simulink model "R_Mode_v1"  (R2020a)
settings: Solver=FixedStepAuto  StartTime=0.0  StopTime=10.0  FixedStep=1e-3  RelTol=1e-3  EnableMultiTasking=on
undefined symbols (not defined in the file): D0, D1, D10, D11, D12, D13, D2, D3, D4, D5, D6, D7, D8, D9, PTA0, PTA1, PTA2, PTB23, PTB9, PTC16, PTC17, PTC2, PTC3, PTC4, PTD0, PTD1, PTD2, PTD3
libraries: frdmk64flib x23
settings Model: ExtModeTrigDuration=5  Creator=forre  LastModifiedBy=forre
settings OptimizationCC: EnhancedBackFolding=on  PassReuseOutputArgsAs=Individual arguments  ZeroExternalMemoryAtStartup=off  ZeroInternalMemoryAtStartup=off  MaxStackSize=64  OptimizeBlockOrder=speed  DifferentSizesBufferReuse=on  OptimizationCustomize=off  EfficientTunableParamExpr=on
settings DebuggingCC: ParameterTunabilityLossMsg=error
settings HardwareCC: ProdBitPerPointer=32  ProdBitPerSizeT=32  ProdBitPerPtrDiffT=32  ProdLargestAtomicInteger=Long  ProdLargestAtomicFloat=Double  ProdWordSize=32  ProdHWDeviceType=ARM Compatible->ARM Cortex
settings SFSimCC: MATLABDynamicMemAlloc=off
settings RTWCC: SystemTargetFile=ert.tlc  HardwareBoard=NXP FRDM-K64F  TemplateMakefile=ert_default_tmf  Toolchain=GNU Tools for ARM Embedded Processors
settings CodeAppCC: ForceParamTrailComments=on  IgnoreCustomStorageClasses=off  OperatorAnnotations=on  SimulinkDataObjDesc=on  SFDataObjDesc=on  InsertBlockDesc=on

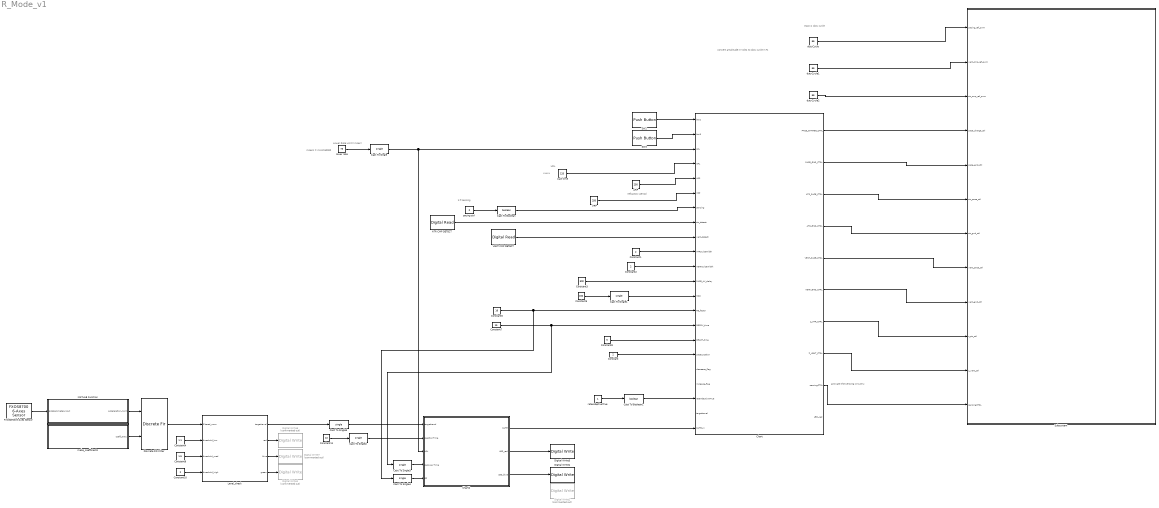
== system R_Mode_v1 ==
  note: convert amplitude in Volts to duty cycle in %
  note: *****
  note: msecs = mins*60000
  note: URL
  note: refractory period
  note: Lower Rate Limit (msec)
  note: activate the sensing circuitry.
  note: input = duty cycle
  note: 1 if sensing
  ARP : Constant  Value=250
  ATR CMP DETECT : frdmk64flib/Digital Read  Whichpin=PTC16 (D0)  SampleTime=-1
  Cast To Boolean : DataTypeConversion  OutDataTypeStr=boolean
  Cast To Boolean1 : DataTypeConversion  OutDataTypeStr=boolean
  Cast To Single{,1..5} (6 alike) : DataTypeConversion  OutDataTypeStr=single
  Chart : Stateflow chart  TreatAsAtomicUnit=on
  Chart2 : Stateflow chart  TreatAsAtomicUnit=on
  Constant : Constant  Value=2  OutDataTypeStr=double
  Constant1 : Constant  Value=2
  Constant10 : Constant  Value=2  OutDataTypeStr=double
  Constant11 : Constant  Value=10  OutDataTypeStr=double
  Constant2 : Constant  Value=2
  Constant3 : Constant  Value=500
  Constant4 : Constant  Value=1.1  OutDataTypeStr=double
  Constant5 : Constant  Value=150  OutDataTypeStr=double
  Constant6 : Constant  Value=16  OutDataTypeStr=double
  Constant7 : Constant  Value=15  OutDataTypeStr=double
  Constant8 : Constant  Value=5  OutDataTypeStr=double
  Constant9 : Constant  Value=1.5  OutDataTypeStr=double
  Digital Write1 : frdmk64flib/Digital Write  Commented=on  Whichpin=GREEN_LED
  Digital Write2 : frdmk64flib/Digital Write  Commented=on  Whichpin=GREEN_LED
  Digital Write3 : frdmk64flib/Digital Write  Whichpin=RED_LED
  Digital Write4 : frdmk64flib/Digital Write  Whichpin=BLUE_LED
  Digital Write6 : frdmk64flib/Digital Write  Commented=on  Whichpin=RED_LED
  Digital Write7 : frdmk64flib/Digital Write  Commented=on  Whichpin=BLUE_LED
  Discrete FIR Filter : DiscreteFir  CoefSource=Input port  Coefficients=[0.05, 0.05, 0.05,0.05, 0.05, 0.05, 0.05, 0.05,0.05, 0.05,0.05, 0.05, 0.05,0.05, 0.05, 0.05, 0.05, 0.05,0.05, 0.05]
      settings: InputPortMap=u0,u1
  FXOS8700 6-Axes Sensor : frdmk64flib/FXOS8700 6-Axes Sensor  Activesensor=Accelerometer only  ODR=800Hz  HybridODR=400Hz  Accelfullrange=-2g to +2g  SampleTime=-1
  Level_check : MATLAB Function  TreatAsAtomicUnit=on
  MATLAB Function : MATLAB Function  TreatAsAtomicUnit=on
  SW2 : frdmk64flib/Push Button  Whichswitch=SW2  SampleTime1=-1
  SW3 : frdmk64flib/Push Button  Whichswitch=SW3  SampleTime1=-1
  Subsystem : Subsystem
  VENT CMP DETECT : frdmk64flib/Digital Read  Whichpin=PTC17 (D1)  SampleTime=-1
  VRP : Constant  Value=250
  dutyCycle : Constant  Value=66
  dutyCycle1 : Constant  Value=66
  dutyCycle2 : Constant  Value=66
  lower rate : Constant  Value=75
  make_coefficients : MATLAB Function  TreatAsAtomicUnit=on
  pacing ctrl : Constant  Value=0
  rateAdaptiveTrue : Constant
  wait time : Constant  Value=120
  wires:
  dutyCycle/1 -> Subsystem/1(pacing_ref_pwm)
  SW2/1 -> Chart/1(btn2)
  Chart/4(ATR_GND_CTRL) -> Subsystem/7(atr_gnd_ctrl)
  Constant1/1 -> Chart/10(ATRpulseWidth)
  Chart/3(ATR_PACE_CTRL) -> Subsystem/6(atr_pace_ctrl)
  Chart/1(PACE_CHARGE_CTRL) -> Subsystem/4(pace_charge_ctrl)
  Chart/2(PACE_GND_CTRL) -> Subsystem/5(pace_gnd_ctrl)
  lower rate/1 -> Cast To Single/1
  Chart/5(VENT_PACE_CTRL) -> Subsystem/8(vent_pace_ctrl)
  Chart/6(VENT_GND_CTRL) -> Subsystem/9(vent_gnd_ctrl)
  Chart/7(Z_ATR_CTRL) -> Subsystem/10(z_atr_ctrl)
  Chart/8(Z_VENT_CTRL) -> Subsystem/11(" z_vent_ctrl")
  pacing ctrl/1 -> Cast To Boolean/1
  ATR CMP DETECT/1 -> Chart/8(atr_detect)
  VENT CMP DETECT/1 -> Chart/9(vent_detect)
  dutyCycle1/1 -> Subsystem/2(vent_cmp_ref_pwm)
  dutyCycle2/1 -> Subsystem/3(atr_cmp_ref_pwm)
  Chart/9(sensingCTRL) -> Subsystem/12(sensingCTRL)
  Cast To Boolean/1 -> Chart/7(sensing)
  Chart2/3(LED_blue) -> Digital Write4/1
  SW3/1 -> Chart/2(btn3)
  wait time/1 -> Chart/4(URL)
  ARP/1 -> Chart/5(ARP)
  VRP/1 -> Chart/6(VRP)
  Constant2/1 -> Chart/11(VENTpulseWidth)
  Constant/1 -> Chart/17(paceLocation)
  Constant3/1 -> Chart/12(PACE_AV_delay)
  Constant5/1 -> Cast To Single1/1
  Constant6/1 -> Chart/14(RE_factor), Cast To Single4/1
  Constant7/1 -> Chart/15(RECOV_time), Cast To Single3/1
  Constant8/1 -> Chart/16(REACT_time)
  Cast To Boolean1/1 -> Chart/20(rateAdaptiveTrue)
  rateAdaptiveTrue/1 -> Cast To Boolean1/1
  Chart2/1(RATE) -> Chart/22(RATE_in)
  Cast To Single/1 -> Chart/3(LRL), Chart2/3(LRL)
  Constant11/1 -> Cast To Single2/1
  Cast To Single1/1 -> Chart/13(MSR)
  Cast To Single2/1 -> Chart2/2(reactionTime)
  Cast To Single3/1 -> Chart2/4(recoveryTime)
  Cast To Single4/1 -> Chart2/5(RF)
  Chart2/2(LED_red) -> Digital Write3/1
  FXOS8700 6-Axes Sensor/1 -> MATLAB Function/1(accelerometer_input)
  Constant4/1 -> Level_check/2(threshold_low)
  Constant10/1 -> Level_check/4(threshold_high)
  Constant9/1 -> Level_check/3(threshold_med)
  Level_check/1(targetLevel) -> Cast To Single5/1
  MATLAB Function/1(acceleration_norm) -> Discrete FIR Filter/1
  Discrete FIR Filter/1 -> Level_check/1(filtered_norm)
  Level_check/2(red) -> Digital Write6/1
  Level_check/3(blue) -> Digital Write7/1
  Level_check/4(green) -> Digital Write1/1
  Cast To Single5/1 -> Chart2/1(targetLevel)
  make_coefficients/1(coeff_array) -> Discrete FIR Filter/2

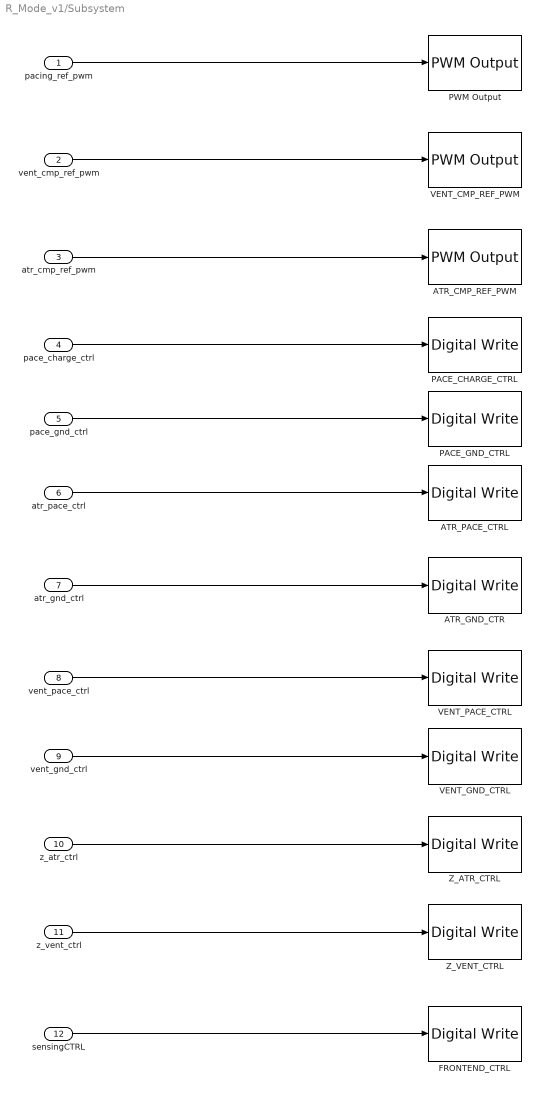
== system R_Mode_v1/Subsystem ==
  pacing_ref_pwm : Inport
  vent_cmp_ref_pwm : Inport  Port=2
  atr_cmp_ref_pwm : Inport  Port=3
  pace_charge_ctrl : Inport  Port=4
  pace_gnd_ctrl : Inport  Port=5
  atr_pace_ctrl : Inport  Port=6
  atr_gnd_ctrl : Inport  Port=7
  vent_pace_ctrl : Inport  Port=8
  vent_gnd_ctrl : Inport  Port=9
  z_atr_ctrl : Inport  Port=10
  " z_vent_ctrl" : Inport  Port=11
  sensingCTRL : Inport  Port=12
  ATR_CMP_REF_PWM : frdmk64flib/PWM Output  Whichpin=PTC2 (D6)  InitialFrequency=2000  InitialDutyCycle=50
  ATR_GND_CTR : frdmk64flib/Digital Write  Whichpin=PTD2 (D11)
  ATR_PACE_CTRL : frdmk64flib/Digital Write  Whichpin=PTA0 (D8)
  FRONTEND_CTRL : frdmk64flib/Digital Write  Whichpin=PTD1 (D13)
  PACE_CHARGE_CTRL : frdmk64flib/Digital Write  Whichpin=PTB9 (D2)
  PACE_GND_CTRL : frdmk64flib/Digital Write  Whichpin=PTD0 (D10)
  PWM Output : frdmk64flib/PWM Output  Whichpin=PTA2 (D5)  InitialFrequency=2000  InitialDutyCycle=50
  VENT_CMP_REF_PWM : frdmk64flib/PWM Output  Whichpin=PTA1 (D3)  InitialFrequency=2000  InitialDutyCycle=50
  VENT_GND_CTRL : frdmk64flib/Digital Write  Whichpin=PTD3 (D12)
  VENT_PACE_CTRL : frdmk64flib/Digital Write  Whichpin=PTC4 (D9)
  Z_ATR_CTRL : frdmk64flib/Digital Write  Whichpin=PTB23 (D4)
  Z_VENT_CTRL : frdmk64flib/Digital Write  Whichpin=PTC3 (D7)
  wires:
  pace_gnd_ctrl/1 -> PACE_GND_CTRL/1
  atr_pace_ctrl/1 -> ATR_PACE_CTRL/1
  pace_charge_ctrl/1 -> PACE_CHARGE_CTRL/1
  atr_gnd_ctrl/1 -> ATR_GND_CTR/1
  vent_pace_ctrl/1 -> VENT_PACE_CTRL/1
  vent_gnd_ctrl/1 -> VENT_GND_CTRL/1
  z_atr_ctrl/1 -> Z_ATR_CTRL/1
  " z_vent_ctrl"/1 -> Z_VENT_CTRL/1
  sensingCTRL/1 -> FRONTEND_CTRL/1
  pacing_ref_pwm/1 -> PWM Output/1
  vent_cmp_ref_pwm/1 -> VENT_CMP_REF_PWM/1
  atr_cmp_ref_pwm/1 -> ATR_CMP_REF_PWM/1

== stateflow chart R_Mode_v1/Chart ==
  note: IF target level > previous level
  note: target Level = LEVEL
  note: if level = 0
      | RATE = LRL
      |
      | if level = 1
      | RATE = LRL + ResponseFactor
      |
      | if level = 2
      | RATE = LRL + 2*ResponseFactor
      |
      | if level = 3
      | RATE = LRL + 3*ResponseFactor
  state INCREMENT_VENT [commented out]
    entry:
    incrementTime=reactionTime/((TargetLevel - PreviousLevel)*RF);
    % time/BPM increase
  note: incrementTime=reactionTime/((TargetLevel - PreviousLevel)*RF)
  state SENSING_VENT_TRUE
    entry:
    sensingCTRL = true;
  note: for VOO,VVI, so it don't go to REACTION_V and RECOVERY_V
  note: ventPflag = true
  state adaptRATE_vent
    % RE factor need to time a rate (unit ppm)
    %it is depend on LRL and MSR values
    %RATE_out = RATE
    RATE = RATE_in;
  note: new Idea!
      |
      | secPerPace = msecPerPace/1000
      |
      | reactionTime/secPerPace = %of increase per cycle
  note: no more change in RATE needed
  note: eg if reactionTIme = 10 and RATE = 60 BPM
      | 10/1 =10
      | incrementAmount = (targetLevel-previousLevel)*RF/10
      |
      | so each cycle RATE = RATE + incrementAmount
  state VENT_CHARGING_AND_DISCHARGE
    entry:
    % for this state paceLocation = 1
    %begin charge and discharge cycle for ventricle
    msecPerPace = 60000.0/RATE/2; %new value in msec
    sensingCTRL = sensing; %enables the sensing circuitry if sensing = 1. Controled by input "sensing"
    ATR_PACE_CTRL = false;
    VENT_PACE_CTRL = false;
    PACE_CHARGE_CTRL = true;
    PACE_GND_CTRL = true;
    Z_VENT_CTRL = false;
    Z_ATR_CTRL = false
    VENT_GND_CTRL = true;
    ATR_GND_CTRL = false;
  state VENT_PACING
    entry:
    % pace ventricle
    PACE_CHARGE_CTRL = false;
    PACE_GND_CTRL = true;
    VENT_PACE_CTRL = true;
    VENT_GND_CTRL = false;
    Z_VENT_CTRL = false;
    Z_ATR_CTRL = false;
    ATR_GND_CTRL = false;
    ATR_PACE_CTRL = false;
    sensingCTRL = sensing; %enables the sensing circuitry if sensing = 1. Controled by input "sensing"
    %VENT_P_flag = true; %pacing flag for V modes
    %recovery
    %recoveryTime_remaining = recoveryTime_remaining - (msecPerPace-VENTpulseWidth)
    LED_red=false;
  note: reactionTime_remaining
  note: recoveryTime_remaining
  note: beat sensed
  note: R_MODE
  note: VENT PACING
  note: SWITCH TO VOO,VVI,VOOR,VVIR
  state RECOVERY_V [commented out]
    RATE = RATE - LEVEL*RE_factor
    % RE factor need to time a rate (unit ppm)
    %it is depend on LRL and MSR values
  state REACTION_V [commented out]
    RATE = RATE + LEVEL*RE_factor;
    % RE factor need to time a rate (unit ppm)
    %it is depend on LRL and MSR values
  note: SWITCH TO AOO, AAI,AOOR,AAIR
  state ATR_PACING [commented out]
    entry:
    % pace atrium
    PACE_GND_CTRL = true;
    VENT_PACE_CTRL = false;
    VENT_GND_CTRL = false;
    Z_VENT_CTRL = false;
    Z_ATR_CTRL = false;
    ATR_GND_CTRL = false;
    ATR_PACE_CTRL = true;
    sensingCTRL = sensing; %enables the sensing circuitry if sensing = 1. Controled by input "sensing"
    ATR_P_flag = true; %pacing flag for V modes
  note: SWITCH TO DOO,DOOR
  state ATR_CHARGING_AND_DISCHARGE [commented out]
    entry:
    % for this state paceLocation = 0
    %begin charge and discharge cycle for atrium
    msecPerPace = 60000/RATE; %new value for pace timing with msec units
    sensingCTRL = sensing; %enables the sensing circuitry if sensing = 1. Controled by input "sensing"
    ATR_PACE_CTRL = false;
    VENT_PACE_CTRL = false;
    PACE_CHARGE_CTRL = true;
    PACE_GND_CTRL = true;
    Z_VENT_CTRL = false;
    Z_ATR_CTRL = false;
    VENT_GND_CTRL = false;
    ATR_GND_CTRL = true;
  note: R_MODE
  note: ATR PACING
  note: SWITCH TO VOO,VVI,VOOR,VVIR
  state SENSING_ATR_TRUE [commented out]
    entry:
    sensingCTRL = true;
  note: beat sensed
  note: SWITCH TO DOO,DOOR
  state RECOVERY_V1 [commented out]
    RATE = RATE - LEVEL*RE_factor
    % RE factor need to time a rate (unit ppm)
    %it is depend on LRL and MSR values
  note: SWITCH TO AOO, AAI,AOOR,AAIR
  state REACTION_V1 [commented out]
    RATE = RATE + LEVEL*RE_factor;
    % RE factor need to time a rate (unit ppm)
    %it is depend on LRL and MSR values
  state DUAL_ATR_CHARGING_AND_DISCHARGE [commented out]
    entry:
    msecPerPace = 60000/RATE;
    % for this state paceLocation = 3
    %begin charge and discharge cycle for atrium
    ATR_PACE_CTRL = false;
    VENT_PACE_CTRL = false;
    PACE_CHARGE_CTRL = true;
    PACE_GND_CTRL = true;
    Z_VENT_CTRL = false;
    Z_ATR_CTRL = false;
    VENT_GND_CTRL = false;
    ATR_GND_CTRL = true;
  state DUAL_ATR_PACING [commented out]
    entry:
    % pace atrium
    PACE_GND_CTRL = true;
    VENT_PACE_CTRL = false;
    VENT_GND_CTRL = false;
    Z_VENT_CTRL = false;
    Z_ATR_CTRL = false;
    ATR_GND_CTRL = false;
    ATR_PACE_CTRL = true;
    AP_flag = true; % rise to true when Atrium have a pace
  note: DOO,DOOR
  state DUAL_VENT_PACING [commented out]
    entry:
    % pace ventricle
    PACE_GND_CTRL = true;
    VENT_PACE_CTRL = true;
    VENT_GND_CTRL = false;
    Z_VENT_CTRL = false;
    Z_ATR_CTRL = false;
    ATR_GND_CTRL = false;
    ATR_PACE_CTRL = false;
    sensingCTRL = sensing; %enables the sensing circuitry if sensing = 1. Controled by input "sensing"
    AP_flag = false;
  state DUAL_VENT_CHARGING_AND_DISCHARGE [commented out]
    entry:
    %begin charge and discharge cycle for ventricle
    msecPerPace = 60000/RATE; %new value in msec
    sensingCTRL = sensing; %enables the sensing circuitry if sensing = 1. Controled by input "sensing"
    ATR_PACE_CTRL = false;
    VENT_PACE_CTRL = false;
    PACE_CHARGE_CTRL = true;
    PACE_GND_CTRL = true;
    Z_VENT_CTRL = false;
    Z_ATR_CTRL = false
    VENT_GND_CTRL = true;
    ATR_GND_CTRL = false;
  INCREMENT_VENT -> INCREMENT_VENT [commented out] : after(incrementTime)[reactionTime_remaining>0]{RATE=RATE+1;reactionTime_remaining-incrementTime;}
  (junction 296) -> VENT_CHARGING_AND_DISCHARGE [order 1] : [rateAdaptiveTrue == false]{RATE=LRL}
  VENT_CHARGING_AND_DISCHARGE -> SENSING_VENT_TRUE [order 2] : after((VRP-VENTpulseWidth),msec)[sensing && (vent_detect || btn3)]
  SENSING_VENT_TRUE -> VENT_CHARGING_AND_DISCHARGE : after(VENTpulseWidth, msec)
  INCREMENT_VENT -> INCREMENT_VENT [commented out] : [reactionTime_remaining <= 0]{previousLevel = LEVEL}
  VENT_PACING -> (junction 296) : after(VENTpulseWidth, msec)
  (junction 296) -> adaptRATE_vent [order 2] : [rateAdaptiveTrue == true]
  adaptRATE_vent -> (junction 386) [commented out] : [(decrease_flag == false && increase_flag == false)]
  adaptRATE_vent -> adaptRATE_vent [commented out] : [increase_flag == true && (RATE < MSR)]{RATE = RATE_in;LED_red=true;}
  (junction 386) -> VENT_CHARGING_AND_DISCHARGE [order 1] : [RATE< LRL]{RATE = LRL}
  adaptRATE_vent -> (junction 386)
  (junction 386) -> VENT_CHARGING_AND_DISCHARGE [order 2] : [RATE>MSR]{RATE=MSR}
  (junction 386) -> VENT_CHARGING_AND_DISCHARGE [order 3]
  (default) -> VENT_CHARGING_AND_DISCHARGE : {RATE=LRL;LED_red=false;previousLevel = 0;}
  adaptRATE_vent -> adaptRATE_vent [commented out] : [decrease_flag == true && (RATE > LRL)]{RATE = RATE_in}
  VENT_CHARGING_AND_DISCHARGE -> DUAL_ATR_CHARGING_AND_DISCHARGE [commented out] : [(paceLocation == 3) || (paceLocation == 6)]{RATE=LRL}
  (junction 290) -> VENT_CHARGING_AND_DISCHARGE [commented out]
  DUAL_ATR_CHARGING_AND_DISCHARGE -> (junction 290) [commented out] : [(paceLocation == 2) || (paceLocation == 4)]{RATE=LRL}
  ATR_CHARGING_AND_DISCHARGE -> (junction 290) [commented out] : [(paceLocation == 2) || (paceLocation == 4)]{RATE=LRL}
  VENT_CHARGING_AND_DISCHARGE -> VENT_PACING [order 1] : after((msecPerPace-VENTpulseWidth), msec)
  RECOVERY_V -> ? [commented out] : after(((RECOV_time/RE_factor)*60),sec){VENT_P_flag = false}
  VENT_CHARGING_AND_DISCHARGE -> (junction 361) [commented out] : [(paceLocation==4)&&(VENT_P_flag== true)]
  (junction 361) -> VENT_CHARGING_AND_DISCHARGE [commented out] : [increase_flag == false]{VENT_P_flag = false}
  (junction 322) -> VENT_CHARGING_AND_DISCHARGE [commented out] : [(RATE>=MSR)]{RATE=MSR,VENT_P_flag = false}
  REACTION_V -> VENT_CHARGING_AND_DISCHARGE [commented out] : after((REACT_time/RE_factor),sec){VENT_P_flag = false}
  VENT_CHARGING_AND_DISCHARGE -> ATR_CHARGING_AND_DISCHARGE [commented out] : [(paceLocation == 1)|| (paceLocation == 5)]{RATE=LRL,ATR_P_flag = false}
  (junction 366) -> ? [commented out] : [(RATE<=LRL)]{RATE = LRL,VENT_P_flag = false}
  (default) -> (junction 326) [commented out] : [(paceLocation==4)&&(VENT_P_flag== true)]
  (junction 326) -> ? [commented out] : [decrease_flag == false]{VENT_P_flag = false}
  (junction 361) -> (junction 322) [commented out] : [increase_flag == true]
  (junction 326) -> (junction 366) [commented out] : [decrease_flag == true]
  (junction 366) -> RECOVERY_V [commented out] : [(RATE>LRL)]
  (junction 322) -> REACTION_V [commented out] : [RATE<MSR]
  (junction 347) -> ATR_CHARGING_AND_DISCHARGE [commented out] : [paceLocation == 1]{ATR_P_flag = false}
  ATR_PACING -> (junction 347) [commented out] : after(ATRpulseWidth, msec)
  (junction 347) -> ATR_CHARGING_AND_DISCHARGE [commented out] : [paceLocation == 5]
  ATR_CHARGING_AND_DISCHARGE -> (junction 282) [commented out] : [(paceLocation == 3) || (paceLocation == 6)]{RATE=LRL}
  ATR_CHARGING_AND_DISCHARGE -> (junction 353) [commented out] : [ATR_P_flag == false]
  (junction 353) -> ATR_PACING [commented out] : after((msecPerPace-ATRpulseWidth), msec){PACE_CHARGE_CTRL = false;}
  RECOVERY_V1 -> ATR_CHARGING_AND_DISCHARGE [commented out] : after(((RECOV_time/RE_factor)*60),sec){ATR_P_flag = false}
  REACTION_V1 -> ATR_CHARGING_AND_DISCHARGE [commented out] : after((REACT_time/RE_factor),sec){ATR_P_flag = false}
  (junction 341) -> ATR_CHARGING_AND_DISCHARGE [commented out] : [RATE<=LRL]{RATE = LRL,ATR_P_flag = false}
  (junction 331) -> ATR_CHARGING_AND_DISCHARGE [commented out] : [LEVEL==0]{RATE = LRL,ATR_P_flag = false}
  ATR_CHARGING_AND_DISCHARGE -> (junction 341) [commented out] : [(paceLocation==5)&&(ATR_P_flag== true)]
  ATR_CHARGING_AND_DISCHARGE -> SENSING_ATR_TRUE [commented out] : after((ARP-ATRpulseWidth),msec)[sensing && (atr_detect || btn3)]
  SENSING_ATR_TRUE -> ATR_CHARGING_AND_DISCHARGE [commented out] : after(ATRpulseWidth, msec)
  DUAL_ATR_CHARGING_AND_DISCHARGE -> ATR_CHARGING_AND_DISCHARGE [commented out] : [(paceLocation == 1)|| (paceLocation == 5)]{RATE=LRL,ATR_P_flag == false}
  ATR_CHARGING_AND_DISCHARGE -> (junction 336) [commented out] : [(paceLocation==5)&&(ATR_P_flag== true)]
  (junction 336) -> ATR_CHARGING_AND_DISCHARGE [commented out] : [RATE>=MSR]{RATE=MSR,ATR_P_flag = false}
  (junction 341) -> RECOVERY_V1 [commented out] : [RATE>LRL]
  (junction 336) -> (junction 331) [commented out] : [RATE<MSR]
  (junction 331) -> REACTION_V1 [commented out] : [LEVEL>0]
  (junction 282) -> DUAL_ATR_CHARGING_AND_DISCHARGE [commented out] : {AP_flag == false}
  DUAL_ATR_CHARGING_AND_DISCHARGE -> DUAL_ATR_PACING [commented out] : [AP_flag == false]{PACE_CHARGE_CTRL = false;}
  DUAL_ATR_PACING -> DUAL_ATR_CHARGING_AND_DISCHARGE [commented out] : after( ATRpulseWidth, msec)
  DUAL_ATR_CHARGING_AND_DISCHARGE -> (junction 285) [commented out] : [AP_flag == true]
  (junction 285) -> DUAL_VENT_CHARGING_AND_DISCHARGE [commented out] : after(PACE_AV_delay-ATRpulseWidth,msec)
  (junction 288) -> DUAL_ATR_CHARGING_AND_DISCHARGE [commented out] : [AP_flag == false]
  DUAL_VENT_PACING -> DUAL_VENT_CHARGING_AND_DISCHARGE [commented out] : after((VENTpulseWidth), msec)
  DUAL_VENT_CHARGING_AND_DISCHARGE -> DUAL_VENT_PACING [commented out] : [AP_flag == true]{PACE_CHARGE_CTRL = false;}
  DUAL_VENT_CHARGING_AND_DISCHARGE -> (junction 288) [commented out] : after(msecPerPace-VENTpulseWidth-PACE_AV_delay,msec)
  data: PACE_CHARGE_CTRL output boolean; PACE_GND_CTRL output boolean; btn2 input boolean; btn3 input boolean; ATR_PACE_CTRL output boolean; ATR_GND_CTRL output boolean; LRL input single; URL input double; ARP input double; VRP input double; VENT_PACE_CTRL output boolean; VENT_GND_CTRL output boolean; Z_ATR_CTRL output boolean; Z_VENT_CTRL output boolean; sensing input boolean; atr_detect input boolean; vent_detect input boolean; sensingCTRL output boolean; msecPerPace local single; ATRpulseWidth input double; VENTpulseWidth input double; PACE_AV_delay input double; AP_flag local boolean; MSR input single; RE_factor input double; RECOV_time input double; REACT_time input double; paceLocation input double; ATR_P_flag local boolean; VENT_P_flag local boolean; decrease_flag input boolean; increase_flag input boolean; rateAdaptiveTrue input boolean; LED_red output boolean; targetLevel input single; previousLevel local single; RATE local single; RATE_in input single
  data atr_detect settings: description=|
      | 0 = pace atrium
      | 1 = pace ventricle
  data vent_detect settings: description=|
      | 0 = pace atrium
      | 1 = pace ventricle
  data paceLocation settings: description=|
      | 0 = pace atrium
      | 1 = pace ventricle

== stateflow chart R_Mode_v1/Chart2 ==
  note: if level = 0
      | RATE = LRL
      |
      | if level = 1
      | RATE = LRL + ResponseFactor
      |
      | if level = 2
      | RATE = LRL + 2*ResponseFactor
      |
      | if level = 3
      | RATE = LRL + 3*ResponseFactor
  state START
    entry:
    reactionTime_remaining = reactionTime;
    recoveryTime_remaining = recoveryTime;
    LED_red = false;
    LED_blue = false;
    LED_green = false;
  note: incrementTime=reactionTime/((TargetLevel - PreviousLevel)*RF)
  note: IF target level < previous level
  note: decrease
  note: IF target level > previous level
  note: Increase
  state INCREMENT
    entry:
    incrementTime=reactionTime/((target - previousLevel)*RF);
    % time/BPM increase
    LED_blue = true;
  state DECREMENT
    entry:
    decrementTime=recoveryTime/((previousLevel - target)*RF);
    % time/BPM increase
    LED_red = true;
  note: [RATE<RATE+(target-previousLevel)]{RATE+RF}
  (default) -> START : {previousLevel = 0;RATE=LRL;}
  START -> INCREMENT [order 1] : [targetLevel > previousLevel]{target = targetLevel}
  START -> DECREMENT [order 2] : [targetLevel < previousLevel]{target = targetLevel}
  INCREMENT -> START [order 1] : [reactionTime_remaining <= 0]{previousLevel = target}
  INCREMENT -> START [order 3] : [targetLevel <= previousLevel]{previousLevel = target}
  DECREMENT -> START [order 3] : [targetLevel >= previousLevel]{previousLevel = target}
  DECREMENT -> START [order 1] : [recoveryTime_remaining <= 0]{previousLevel = target}
  DECREMENT -> DECREMENT [order 2] : after(decrementTime, sec)[recoveryTime_remaining>0]{RATE=RATE-1;recoveryTime_remaining=recoveryTime_remaining-decrementTime;}
  INCREMENT -> INCREMENT [order 2] : after(incrementTime,sec)[reactionTime_remaining>0]{RATE=RATE+1;reactionTime_remaining=reactionTime_remaining-incrementTime;}
  data: targetLevel input single; reactionTime input single; RATE output single; LRL input single; previousLevel local single; recoveryTime input single; decrementTime local single; incrementTime local single; reactionTime_remaining local single; recoveryTime_remaining local single; RF input single; LED_red output boolean; LED_blue output boolean; target local single

== matlab function R_Mode_v1/MATLAB Function ==
  data: accelerometer_input input; acceleration_norm output
function acceleration_norm = fcn(accelerometer_input)
acceleration_norm = sqrt((accelerometer_input(1))^2+(accelerometer_input(2))^2+(accelerometer_input(3))^2);

== matlab function R_Mode_v1/Level_check ==
  data: filtered_norm input; targetLevel output; threshold_low input; threshold_med input; threshold_high input; red output; blue output; green output
function [targetLevel, red, blue, green] = fcn(filtered_norm,threshold_low,threshold_med,threshold_high)
red = false;
blue = false;
green = false;

if filtered_norm >= threshold_high
    targetLevel = 3;
    red = true;

elseif filtered_norm >= threshold_med
    targetLevel = 2;
    green = true;
    
elseif filtered_norm >= threshold_low
    targetLevel = 1;
    blue = true;
    
else
    targetLevel = 0;
    
    red = false;
    blue = false;
    green = false;
end

== matlab function R_Mode_v1/make_coefficients ==
  data: coeff_array output double
function coeff_array = fcn()
coeff_array= ones(500,1)/500;
